simulink model "Lib"  (R2022a)
settings: Solver=VariableStepAuto  StartTime=0.0  StopTime=10.0  RelTol=1e-3
libraries: simulink x3
settings Model: Creator=Castiel  LastModifiedBy=JSF

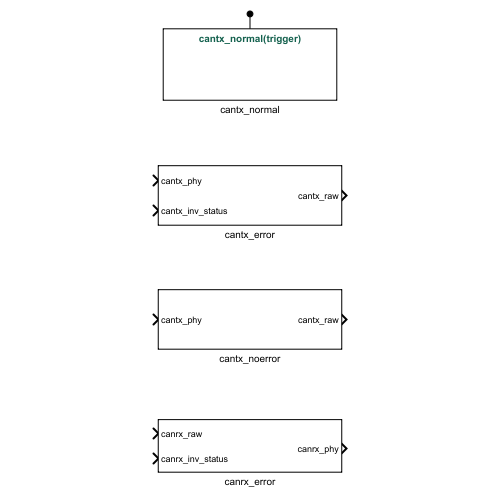
[thumbnail: Simulink's stored preview of the top-level diagram]
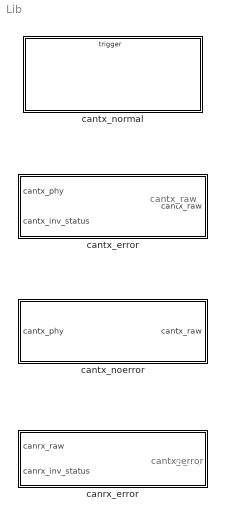
== system Lib ==
  note: cantx_error
  note: cantx_raw
  canrx_error : Subsystem
  cantx_error : Subsystem
  cantx_noerror : Subsystem
  cantx_normal : Subsystem  TreatAsAtomicUnit=on

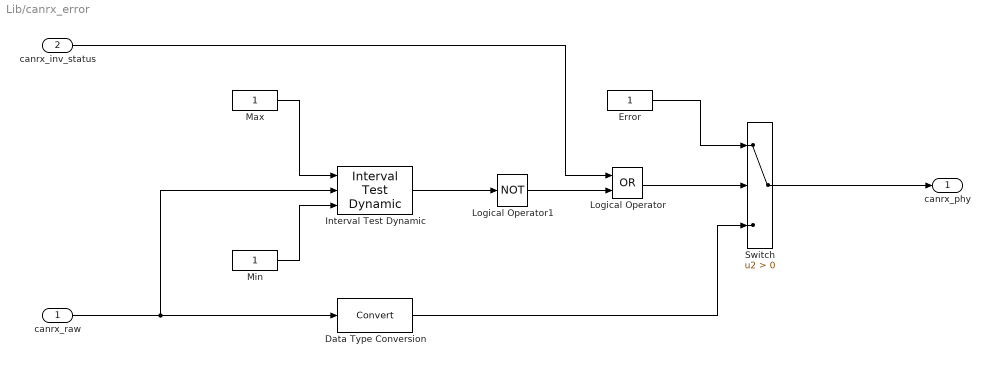
== system Lib/canrx_error ==
  canrx_raw : Inport
  canrx_inv_status : Inport  Port=2
  Data Type Conversion : DataTypeConversion  SaturateOnIntegerOverflow=off  RndMeth=Floor
  Error : Constant  OutDataTypeStr=Inherit: Inherit via back propagation
  Interval Test Dynamic : simulink/Logic and Bit Operations/Interval Test Dynamic  IntervalClosedRight=on  IntervalClosedLeft=on  OutDataTypeStr=boolean
  Logical Operator : Logic  Operator=OR  AllPortsSameDT=off  OutDataTypeStr=boolean
  Logical Operator1 : Logic  Operator=NOT  AllPortsSameDT=off  OutDataTypeStr=boolean
  Max : Constant  OutDataTypeStr=Inherit: Inherit via back propagation
  Min : Constant  OutDataTypeStr=Inherit: Inherit via back propagation
  Switch : Switch  Criteria=u2 > Threshold  SaturateOnIntegerOverflow=off  InputSameDT=off
  canrx_phy : Outport
  wires:
  canrx_raw/1 -> Data Type Conversion/1, Interval Test Dynamic/2
  Max/1 -> Interval Test Dynamic/1
  Min/1 -> Interval Test Dynamic/3
  Data Type Conversion/1 -> Switch/3
  Interval Test Dynamic/1 -> Logical Operator1/1
  Logical Operator1/1 -> Logical Operator/2
  canrx_inv_status/1 -> Logical Operator/1
  Logical Operator/1 -> Switch/2
  Error/1 -> Switch/1
  Switch/1 -> canrx_phy/1

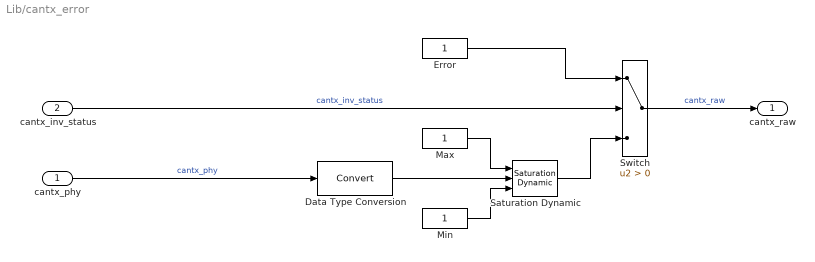
== system Lib/cantx_error ==
  cantx_phy : Inport
  cantx_inv_status : Inport  Port=2
  Data Type Conversion : DataTypeConversion  SaturateOnIntegerOverflow=off  RndMeth=Floor
  Error : Constant  OutDataTypeStr=Inherit: Inherit via back propagation
  Max : Constant  OutDataTypeStr=Inherit: Inherit via back propagation
  Min : Constant  OutDataTypeStr=Inherit: Inherit via back propagation
  Saturation Dynamic : simulink/Discontinuities/Saturation Dynamic  OutMin=[]  OutMax=[]  OutDataTypeStr=Inherit: Same as second input  OutDataType=fixdt(1, 16)  OutScaling=2^-10  DoSatur=off
  Switch : Switch  Criteria=u2 > Threshold  SaturateOnIntegerOverflow=off  InputSameDT=off
  cantx_raw : Outport
  wires:
  cantx_inv_status/1 -> Switch/2  "cantx_inv_status"
  Max/1 -> Saturation Dynamic/1
  Error/1 -> Switch/1
  Min/1 -> Saturation Dynamic/3
  cantx_phy/1 -> Data Type Conversion/1  "cantx_phy"
  Data Type Conversion/1 -> Saturation Dynamic/2
  Saturation Dynamic/1 -> Switch/3
  Switch/1 -> cantx_raw/1  "cantx_raw"

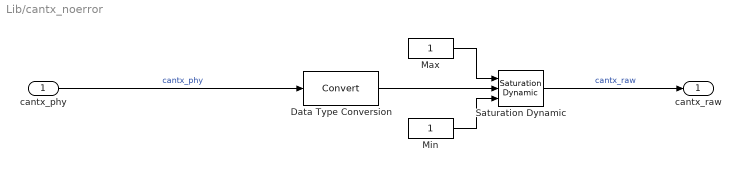
== system Lib/cantx_noerror ==
  cantx_phy : Inport
  Data Type Conversion : DataTypeConversion  SaturateOnIntegerOverflow=off  RndMeth=Floor
  Max : Constant  OutDataTypeStr=Inherit: Inherit via back propagation
  Min : Constant  OutDataTypeStr=Inherit: Inherit via back propagation
  Saturation Dynamic : simulink/Discontinuities/Saturation Dynamic  OutMin=[]  OutMax=[]  OutDataTypeStr=Inherit: Same as second input  OutDataType=fixdt(1, 16)  OutScaling=2^-10  DoSatur=off
  cantx_raw : Outport
  wires:
  Max/1 -> Saturation Dynamic/1
  Min/1 -> Saturation Dynamic/3
  cantx_phy/1 -> Data Type Conversion/1  "cantx_phy"
  Data Type Conversion/1 -> Saturation Dynamic/2
  Saturation Dynamic/1 -> cantx_raw/1  "cantx_raw"

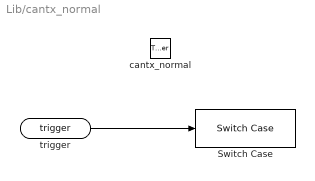
== system Lib/cantx_normal ==
  cantx_normal : TriggerPort  TriggerType=function-call  IsSimulinkFunction=on  FunctionName=cantx_normal  FunctionVisibility=scoped  VariantControl=(inherit)
  Switch Case : SwitchCase  CaseConditions={0}  ShowDefaultCase=off
  trigger : ArgIn  DisableCoverage=on  ArgumentName=trigger
  wires:
  trigger/1 -> Switch Case/1
